simulink model "ejercicio_puntos"  (R2018a)
settings: Solver=VariableStepAuto  StartTime=0.0  StopTime=10.0  RelTol=1e-3
settings Model: Creator=hanan  LastModifiedBy=hanan

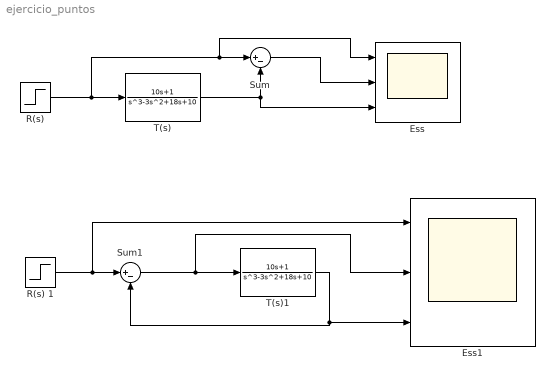
== system ejercicio_puntos ==
  "Ess " : Scope  NumInputPorts=3
  Ess1 : Scope  NumInputPorts=3
  "R(s) " : Step  SampleTime=0
  R(s) 1 : Step  SampleTime=0
  Sum : Sum  Inputs=|+-
  Sum1 : Sum  Inputs=|+-
  T(s) : TransferFcn  Numerator=[10 1]  Denominator=[1 -3 18 10]
  T(s)1 : TransferFcn  Numerator=[10 1]  Denominator=[1 -3 18 10]
  wires:
  "R(s) "/1 -> "Ess "/1, Sum/1, T(s)/1
  T(s)/1 -> Sum/2, "Ess "/3
  Sum1/1 -> Ess1/2, T(s)1/1
  R(s) 1/1 -> Ess1/1, Sum1/1
  T(s)1/1 -> Sum1/2, Ess1/3
  Sum/1 -> "Ess "/2
